simulink model "AEBS"  (R2022b)
settings: configuration reference "CommonModelConfiguration" (kept outside this file)
undefined symbols (not defined in the file): cc_param_311, cc_param_369, LCFG_ACPE_Timeout, LCFG_AEBS_SignalTimeout
settings Model: Creator=JELIASS5  LastModifiedBy=AJOSHI11
settings ConfigSetRef: SourceName=CommonModelConfiguration  SourceLocation=Base Workspace

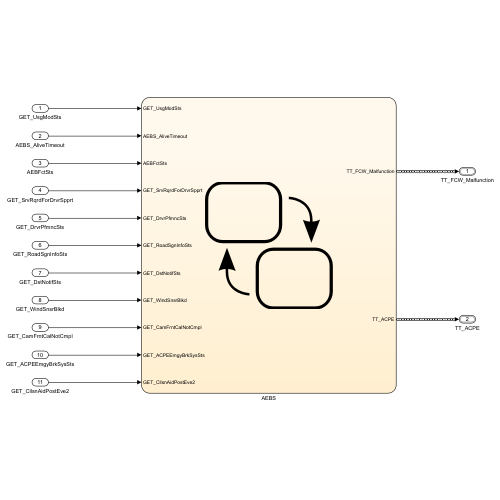
[thumbnail: Simulink's stored preview of the top-level diagram]
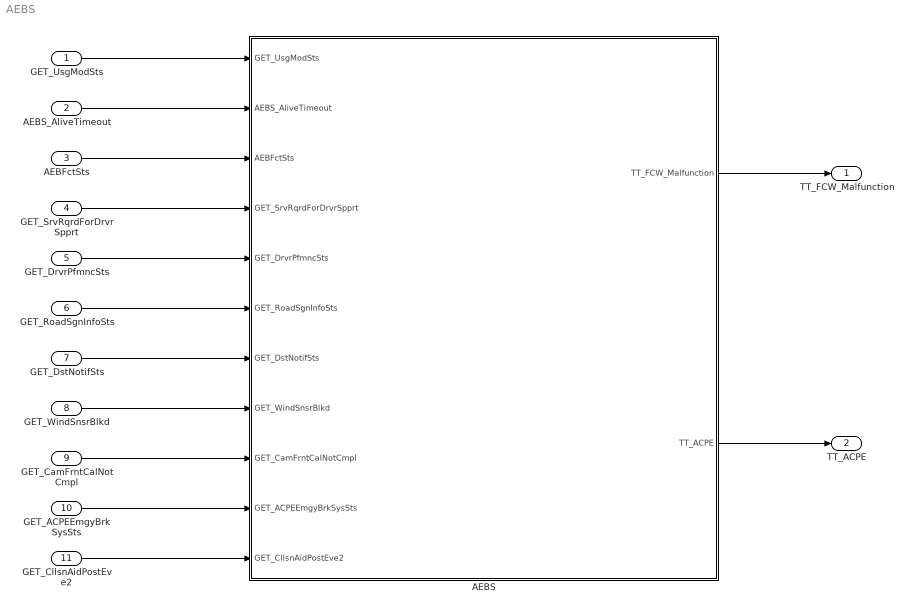
== system AEBS ==
  GET_UsgModSts : Inport  OutDataTypeStr=Enum: UsgModSts1
  AEBS_AliveTimeout : Inport  Port=2  OutDataTypeStr=boolean
  AEBFctSts : Inport  Port=3  OutDataTypeStr=Enum: UkwnOffOn
  GET_SrvRqrdForDrvrSpprt : Inport  Port=4  OutDataTypeStr=Enum: OnOff1
  GET_DrvrPfmncSts : Inport  Port=5  OutDataTypeStr=Enum: FctSts2
  GET_RoadSgnInfoSts : Inport  Port=6  OutDataTypeStr=Enum: FctSts2
  GET_DstNotifSts : Inport  Port=7  OutDataTypeStr=Enum: FctSts2
  GET_WindSnsrBlkd : Inport  Port=8  OutDataTypeStr=Enum: OnOff1
  GET_CamFrntCalNotCmpl : Inport  Port=9  OutDataTypeStr=Enum: NoYes1
  GET_ACPEEmgyBrkSysSts : Inport  Port=10  OutDataTypeStr=Enum: ACPEEmgyBrkSysSts  LockScale=on
  GET_CllsnAidPostEve2 : Inport  Port=11  OutDataTypeStr=Enum: CllsnAidPostEve3  LockScale=on
  AEBS : Stateflow chart  TreatAsAtomicUnit=on
  TT_FCW_Malfunction : Outport  OutDataTypeStr=Bus: PA_StatusAndOffOnChinaValue  VectorParamsAs1DForOutWhenUnconnected=off
  TT_ACPE : Outport  Port=2  OutDataTypeStr=Bus: PA_StatusAndOffOnChinaValue  VectorParamsAs1DForOutWhenUnconnected=off
  wires:
  AEBS/1(TT_FCW_Malfunction) -> TT_FCW_Malfunction/1
  GET_UsgModSts/1 -> AEBS/1(GET_UsgModSts)
  AEBS_AliveTimeout/1 -> AEBS/2(AEBS_AliveTimeout)
  AEBFctSts/1 -> AEBS/3(AEBFctSts)
  GET_SrvRqrdForDrvrSpprt/1 -> AEBS/4(GET_SrvRqrdForDrvrSpprt)
  GET_DrvrPfmncSts/1 -> AEBS/5(GET_DrvrPfmncSts)
  GET_RoadSgnInfoSts/1 -> AEBS/6(GET_RoadSgnInfoSts)
  GET_DstNotifSts/1 -> AEBS/7(GET_DstNotifSts)
  GET_WindSnsrBlkd/1 -> AEBS/8(GET_WindSnsrBlkd)
  GET_CamFrntCalNotCmpl/1 -> AEBS/9(GET_CamFrntCalNotCmpl)
  GET_CllsnAidPostEve2/1 -> AEBS/11(GET_CllsnAidPostEve2)
  GET_ACPEEmgyBrkSysSts/1 -> AEBS/10(GET_ACPEEmgyBrkSysSts)
  AEBS/2(TT_ACPE) -> TT_ACPE/1

== stateflow chart AEBS/AEBS ==
  state SYSTEM_OK
    state isActive = activationCheck [function]
      (default) -> (junction 34)
      (junction 34) -> (junction 35) [order 1] : %Engine running
          | [GET_UsgModSts==UsgModSts1.UsgModSts1_UsgModDrvg]
      (junction 34) -> (junction 36) [order 2] : {isActive = false;}
      (junction 35) -> (junction 37) : {isActive = true;}
      (junction 37) -> (junction 36)
      (junction 36) -> (junction 57)
    state NOT_ACTIVE
      entry:
      TT_FCW_Malfunction.Status = E_CommonStatus.Disabled;
      TT_FCW_Malfunction.Value = E_OffOnChina.Off;
      TT_ACPE.Value = E_OffOnChina.Off;
      (default) -> (junction 135)
      (junction 135) -> (junction 136) [order 1] : %Argus3
          | [cc_param_311==3]
      (junction 135) -> (junction 141) [order 2] : %ACPE not present
          | {TT_ACPE.Status =...
          | E_CommonStatus.NotPresent}
      (junction 136) -> (junction 139) : %ACPE present but disabled
          | {TT_ACPE.Status =...
          | E_CommonStatus.Disabled;}
      (junction 139) -> (junction 141)
      (junction 141) -> (junction 146)
    state ACTIVE
      state ACPE [parallel]
        settings: executionOrder=1
        state ACPE_ON
          state ON
            en, du:
            TT_ACPE.Value = E_OffOnChina.On;
          state ON_CHINA
            en, du:
            TT_ACPE.Value = E_OffOnChina.On_China;
          (default) -> (junction 115)
          (junction 115) -> SYSTEM_OK.ACTIVE.ACPE.ACPE_ON.ON [order 2]
          (junction 115) -> (junction 118) [order 1] : %China market
              | [cc_param_369==2]
          (junction 118) -> SYSTEM_OK.ACTIVE.ACPE.ACPE_ON.ON_CHINA
        state ACPE_OFF
          en, du:
          TT_ACPE.Status = E_CommonStatus.Available;
          TT_ACPE.Value = E_OffOnChina.Off;
        state ACPE_NOT_PRESENT
          en, du:
          TT_ACPE.Status = E_CommonStatus.NotPresent;
          TT_ACPE.Value = E_OffOnChina.Off;
        (default) -> (junction 129)
        ACPE_OFF -> ACPE_ON : [hasChangedTo(GET_CllsnAidPostEve2, CllsnAidPostEve3.CllsnAidPostEveArgus3_AcpeFrwd) ||...
            | hasChangedTo(GET_CllsnAidPostEve2, CllsnAidPostEve3.CllsnAidPostEveArgus3_AcpeRrwd)]
        (junction 129) -> ACPE_OFF [order 1] : %Argus3
            | [cc_param_311==3]
        (junction 129) -> (junction 130) [order 2]
        ACPE_ON -> ACPE_OFF : [after(LCFG_ACPE_Timeout, sec)]
        (junction 130) -> ACPE_NOT_PRESENT
      state MALFUNCTION [parallel]
        entry: TT_FCW_Malfunction.Status = E_CommonStatus.Available
        settings: executionOrder=2
        state OFF
          en, du:
          TT_FCW_Malfunction.Value = E_OffOnChina.Off;
        state FAULT_ACTIVE
          state ON
            en, du:
            TT_FCW_Malfunction.Value = E_OffOnChina.On;
          state ON_CHINA
            en, du:
            TT_FCW_Malfunction.Value = E_OffOnChina.On_China;
          (default) -> (junction 94)
          (junction 94) -> SYSTEM_OK.ACTIVE.MALFUNCTION.FAULT_ACTIVE.ON [order 2]
          (junction 94) -> (junction 99) [order 1] : %China market
              | [cc_param_369==2]
          (junction 99) -> SYSTEM_OK.ACTIVE.MALFUNCTION.FAULT_ACTIVE.ON_CHINA
        state ALIVE_TIMEOUT
        (default) -> OFF
        OFF -> FAULT_ACTIVE [order 2] : %AEB function unavailable, telltale activated
            | [AEBFctSts==UkwnOffOn.UkwnOffOn_Off ||...
            | GET_WindSnsrBlkd==OnOff1.OnOff1_On ||...
            | GET_CamFrntCalNotCmpl==NoYes1.NoYes1_Yes ||...
            | GET_DrvrPfmncSts==FctSts2.FctSts2_SrvRqrd ||...
            | GET_DstNotifSts==FctSts2.FctSts2_SrvRqrd ||...
            | GET_RoadSgnInfoSts==FctSts2.FctSts2_SrvRqrd ||...
            | GET_SrvRqrdForDrvrSpprt==OnOff1.OnOff1_On ||...
            | (cc_param_311==3 &&...
            | GET_ACPEEmgyBrkSysSts==ACPEEmgyBrkSysSts.ACPEEmgyBrkSysSts_Failure)]
        FAULT_ACTIVE -> OFF : %AEB function available & no AliveTimeout, telltale deactivated
            | [AEBFctSts==UkwnOffOn.UkwnOffOn_On &&...
            | GET_WindSnsrBlkd==OnOff1.OnOff1_Off &&...
            | GET_CamFrntCalNotCmpl==NoYes1.NoYes1_No &&...
            | GET_DrvrPfmncSts~=FctSts2.FctSts2_SrvRqrd &&...
            | GET_DstNotifSts~=FctSts2.FctSts2_SrvRqrd &&...
            | GET_RoadSgnInfoSts~=FctSts2.FctSts2_SrvRqrd &&...
            | GET_SrvRqrdForDrvrSpprt==OnOff1.OnOff1_Off &&...
            | (GET_ACPEEmgyBrkSysSts~=ACPEEmgyBrkSysSts.ACPEEmgyBrkSysSts_Failure && cc_param_311==3) &&...
            | AEBS_AliveTimeout==false]
        OFF -> ALIVE_TIMEOUT [order 1] : [AEBS_AliveTimeout==true]
        ALIVE_TIMEOUT -> OFF [order 1] : [AEBS_AliveTimeout==false]
        ALIVE_TIMEOUT -> FAULT_ACTIVE [order 2] : %After LCFG timer has elapsed OR function becomes unavailable
            | [after(LCFG_AEBS_SignalTimeout, sec) || AEBFctSts==OnOff1.OnOff1_Off]
    (default) -> (junction 26)
    (junction 26) -> NOT_ACTIVE [order 1] : [~activationCheck()]
    (junction 26) -> (junction 29) [order 2]
    NOT_ACTIVE -> ACTIVE : [activationCheck()]
    ACTIVE -> NOT_ACTIVE : [~activationCheck()]
    (junction 29) -> ACTIVE
  data: isActive function_output boolean; TT_FCW_Malfunction output Bus: PA_StatusAndOffOnChinaValue; GET_UsgModSts input Enum: UsgModSts1; AEBS_AliveTimeout input boolean; AEBFctSts input Enum: UkwnOffOn; LCFG_AEBS_SignalTimeout parameter uint8; GET_SrvRqrdForDrvrSpprt input Enum: OnOff1; GET_DrvrPfmncSts input Enum: FctSts2; GET_RoadSgnInfoSts input Enum: FctSts2; GET_DstNotifSts input Enum: FctSts2; GET_WindSnsrBlkd input Enum: OnOff1; GET_CamFrntCalNotCmpl input Enum: NoYes1; GET_ACPEEmgyBrkSysSts input; cc_param_369 parameter uint8; GET_CllsnAidPostEve2 input; TT_ACPE output Bus: PA_StatusAndOffOnChinaValue; LCFG_ACPE_Timeout parameter double; cc_param_311 parameter uint8
